simulink model "PWM_drive_ckt"  (R2021a)
settings: Solver=VariableStepAuto  StartTime=0.0  StopTime=10.0  RelTol=1e-3
undefined symbols (not defined in the file): magnitude
settings Model: Creator=wwwvi  LastModifiedBy=wwwvi

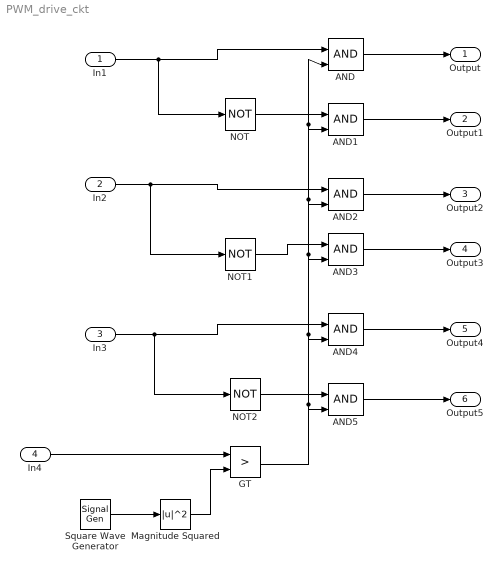
== system PWM_drive_ckt ==
  In1 : Inport
  In2 : Inport  Port=2
  In3 : Inport  Port=3
  In4 : Inport  Port=4
  AND{,1..5} (6 alike) : Logic  IconShape=distinctive  AllPortsSameDT=off  OutDataTypeStr=boolean
  GT : RelationalOperator  Operator=>  OutDataTypeStr=boolean  RndMeth=Simplest
  Magnitude Squared : Math  Operator=magnitude^2  SaturateOnIntegerOverflow=on
  NOT : Logic  Operator=NOT  IconShape=distinctive  AllPortsSameDT=off  OutDataTypeStr=boolean
  NOT1 : Logic  Operator=NOT  IconShape=distinctive  AllPortsSameDT=off  OutDataTypeStr=boolean
  NOT2 : Logic  Operator=NOT  IconShape=distinctive  AllPortsSameDT=off  OutDataTypeStr=boolean
  Square Wave Generator : SignalGenerator  WaveForm=square  Units=rad/sec
  Output : Outport
  Output1 : Outport  Port=2
  Output2 : Outport  Port=3
  Output3 : Outport  Port=4
  Output4 : Outport  Port=5
  Output5 : Outport  Port=6
  wires:
  In1/1 -> NOT/1, AND/1
  In2/1 -> NOT1/1, AND2/1
  In3/1 -> NOT2/1, AND4/1
  NOT/1 -> AND1/1
  NOT1/1 -> AND3/1
  NOT2/1 -> AND5/1
  Square Wave Generator/1 -> Magnitude Squared/1
  In4/1 -> GT/1
  Magnitude Squared/1 -> GT/2
  GT/1 -> AND5/2, AND4/2, AND3/2, AND2/2, AND1/2, AND/2
  AND/1 -> Output/1
  AND1/1 -> Output1/1
  AND2/1 -> Output2/1
  AND3/1 -> Output3/1
  AND4/1 -> Output4/1
  AND5/1 -> Output5/1
